simulink model "InvisibilityCloak"  (R2021b)
settings: Solver=VariableStepAuto  StartTime=0.0  StopTime=50  RelTol=1e-3
undefined symbols (not defined in the file): none, Rec, SDTV, videoinput
libraries: visionconversions x1, imaqlib x1, visionsources x1
settings Model: Creator=mmordeka  LastModifiedBy=mmordeka

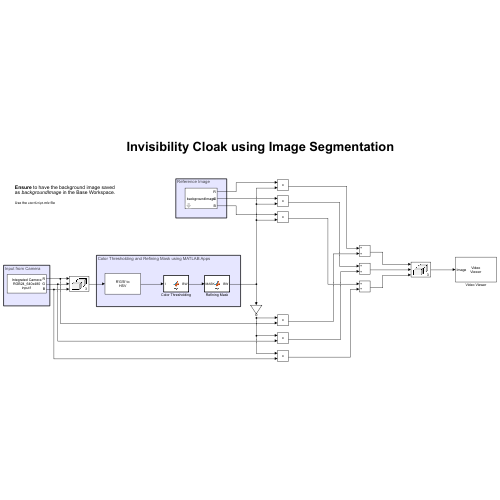
[thumbnail: Simulink's stored preview of the top-level diagram]
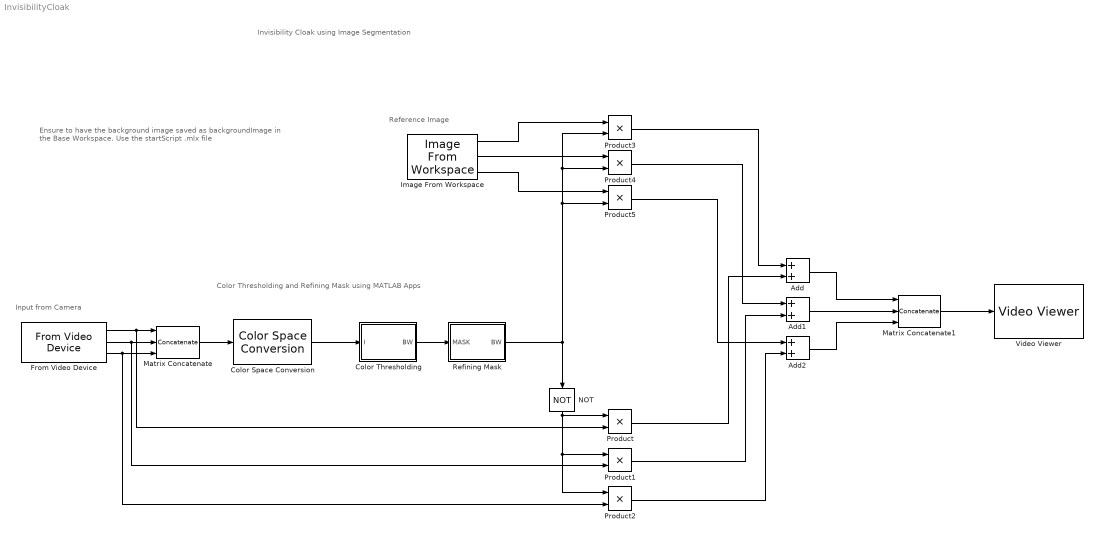
== system InvisibilityCloak ==
  note: Ensure to have the background image saved
      | as backgroundImage in the Base Workspace.
      |
      | Use the startScript .mlx file
  note: Invisibility Cloak using Image Segmentation
  note: Color Thresholding and Refining Mask using MATLAB Apps
  note: Reference Image
  note: Input from Camera
  Add : Sum
  Add1 : Sum
  Add2 : Sum
  Color Space Conversion : visionconversions/Color Space  Conversion  conversion=Obsolete  conversionActive=R'G'B' to HSV  wp_str=D65  rec=Rec. 601 (SDTV)  sys=1125/60/2:1  imagePorts=One multidimensional signal
  Color Thresholding : MATLAB Function  TreatAsAtomicUnit=on
  From Video Device : imaqlib/From Video Device  DeviceMenu=winvideo 1 (Integrated Camera)  Device=winvideo 1 (Integrated Camera)  ObjConstructor=videoinput('winvideo', 1)  VideoFormatMenu=RGB24_640x480  VideoFormat=RGB24_640x480  VideoSource=input1  ROIPosition=[0 0 480 640]  EnableHWTrigger=off  TriggerConfiguration=none/none  SampleTime=1/30  OutputPortsMode=Separate color signals  DataType=single  CanDoHWTrigger=no  ReturnedColorSpace=rgb  BlockHandle=13.0002  ROIWidth=640  ROIHeight=480  ROIColumn=0  ROIRow=0  EngXMLPath=C:\Program Files\MATLAB\R2021b\toolbox\imaq\imaq\private  DevXMLPath=C:\ProgramData\MATLAB\SupportPackages\R2021b\toolbox\imaq\supportpackages\genericvideo\adaptor\win64  EngLibPath=C:\Program Files\MATLAB\R2021b\toolbox\imaq\imaqblks\imaqmex\win64  ColorSpace=rgb  BayerSensorAlignment=grbg  ImaqMode=off
  Image From Workspace : visionsources/Image From Workspace  Tag=vipblks_nd  ImageValue=backgroundImage  Ts=inf  imagePorts=Separate color signals  OutPortLabels=R|G|B  ImageDataType=single  Signed=on  WordLength=16  sdImageDataType=sfix(16)  FractionLengthMode=User-defined  FractionLength=15
      settings: SourceProductBaseCode=VP
  Matrix Concatenate : Concatenate  NumInputs=3  Mode=Multidimensional array  ConcatenateDimension=3
  Matrix Concatenate1 : Concatenate  NumInputs=3  Mode=Multidimensional array  ConcatenateDimension=3
  NOT : Logic  Operator=NOT  IconShape=distinctive  AllPortsSameDT=off  OutDataTypeStr=boolean
  Product{,1..5} (6 alike) : Product
  Refining Mask : MATLAB Function  TreatAsAtomicUnit=on
  Video Viewer : VideoViewer  FigPos=[-1729 1274 1239 681]
  wires:
  Matrix Concatenate/1 -> Color Space Conversion/1
  Color Space Conversion/1 -> Color Thresholding/1(I)
  From Video Device/1 -> Product/2, Matrix Concatenate/1
  From Video Device/2 -> Product1/2, Matrix Concatenate/2
  From Video Device/3 -> Product2/2, Matrix Concatenate/3
  Matrix Concatenate1/1 -> Video Viewer/1
  Image From Workspace/1 -> Product3/1
  Image From Workspace/2 -> Product4/1
  Image From Workspace/3 -> Product5/1
  Color Thresholding/1(BW) -> Refining Mask/1(MASK)
  NOT/1 -> Product/1, Product1/1, Product2/1
  Product3/1 -> Add/1
  Product4/1 -> Add1/1
  Product5/1 -> Add2/1
  Product/1 -> Add/2
  Product1/1 -> Add1/2
  Product2/1 -> Add2/2
  Add2/1 -> Matrix Concatenate1/3
  Add1/1 -> Matrix Concatenate1/2
  Add/1 -> Matrix Concatenate1/1
  Refining Mask/1(BW) -> NOT/1, Product3/2, Product4/2, Product5/2

== matlab function InvisibilityCloak/Color Thresholding ==
  data: I input; BW output
function BW = fcn(I)

channel1Min = 0.02;
channel1Max = 0.098;

% Define thresholds for channel 2 based on histogram settings
channel2Min = 0.662;
channel2Max = 1.000;

% Define thresholds for channel 3 based on histogram settings
channel3Min = 0.395;
channel3Max = 0.851;


% Create mask based on chosen histogram thresholds
sliderBW = (I(:,:,1) >= channel1Min ) & (I(:,:,1) <= channel1Max) & ...
    (I(:,:,2) >= channel2Min ) & (I(:,:,2) <= channel2Max) & ...
    (I(:,:,3) >= channel3Min ) & (I(:,:,3) <= channel3Max);
BW = sliderBW;

== matlab function InvisibilityCloak/Refining Mask ==
  data: MASK input; BW output
function BW = fcn(MASK)

% Create empty mask.
BW = false(size(MASK,1),size(MASK,2));

% Load Mask
BW = MASK;

% Fill holes
BW = imfill(BW, 'holes');

% Open mask with disk
radius = 3;
decomposition = 0;
se = strel('disk', radius, decomposition);
BW = imopen(BW, se);

end
